simulink model "rtwdemo_dow"  (Simulink 7.6)
settings: Solver=FixedStepDiscrete  StartTime=0.0  StopTime=.001  FixedStep=0.001  RelTol=1e-3
PreLoadFcn:
  | rtwdemo_dow_data
values from neighbouring files (symbols this model uses):
  F1 = 2    [rtwdemo_dow_data.m]
  G1 = 4    [rtwdemo_dow_data.m]
  G2 = 5    [rtwdemo_dow_data.m]
  G3 = 6    [rtwdemo_dow_data.m]
  K1 = 3    [rtwdemo_cgv_init.m]    (also in rtwdemo_dow_data.m)
libraries: rtwdemowidgets x2
Description:
  | Creating a Data Dictionary with the Data Object Wizard
settings Model: Creator=The MathWorks Inc.  ExtModeAutoUpdateStatusClock=off
settings MATStruct: SampleTime=0.001  Offset=0  Priority=[20.0]
settings DataIOCC: SaveOutput=off  SaveTime=off
settings OptimizationCC: InlineParams=on  InlineInvariantSignals=on  StateBitsets=on  DataBitsets=on  UseTempVars=on  EfficientFloat2IntCast=on  EfficientMapNaN2IntZero=off  BufferReusableBoundary=off
settings DebuggingCC: CheckExecutionContextPreStartOutputMsg=on  CheckExecutionContextRuntimeOutputMsg=on  SigSpecEnsureSampleTimeMsg=none  StrictBusMsg=ErrorOnBusTreatedAsVector
settings HardwareCC: ProdIntDivRoundTo=Zero  ProdEndianess=LittleEndian  ProdHWDeviceType=Generic->32-bit Embedded Processor  TargetHWDeviceType=Generic->32-bit Embedded Processor
settings SFSimCC: SimParseCustomCode=off
settings RTWCC: GenerateReport=on  RTWVerbose=off  ProcessScript=grt_make_rtw_hook  LaunchReport=on
settings CodeAppCC: ForceParamTrailComments=on
settings GRTTargetCC: TargetFcnLib=ansi_tfl_tmw.mat

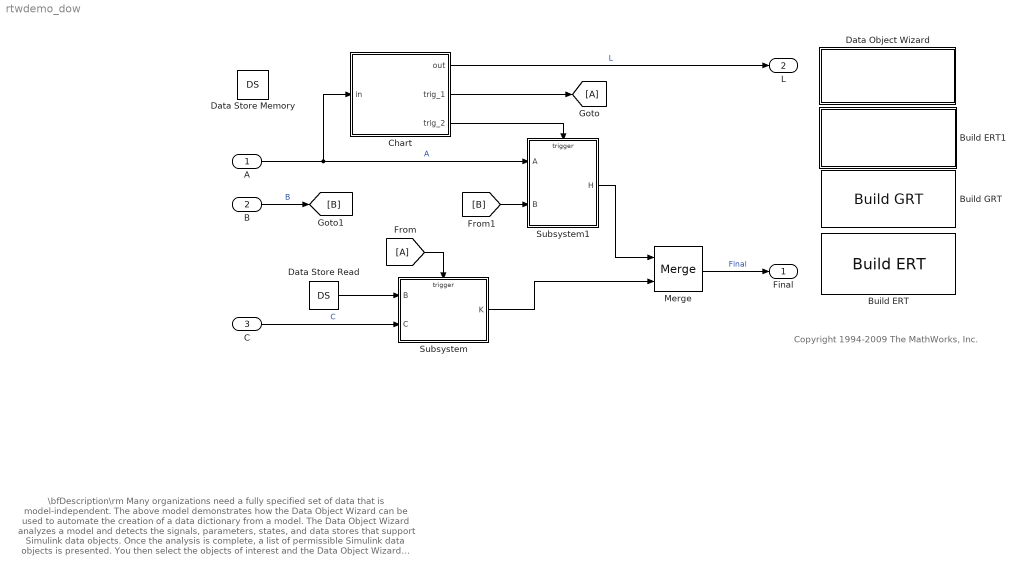
== system rtwdemo_dow ==
  note: \bfDescription\rm
      | Many organizations need a fully specified set of data that is model-independent.  The above model demonstrates how the Data Object Wizard
      | can be used to automate the creation of a data dictionary from a model.  The Data Object Wizard analyzes a model and detects the signals,
      | parameters, states, and data stores that support Simulink data objects.  Once the analysis is complete, a list of permissible Simulink data
      | objects is presented.  You then select the objects of interest and the Data Object Wizard creates the corresponding Simulink data objects.
      |
      | \bfInstructions\rm
      | 1. Double-click the yellow Data Object Wizard button in the upper right of the diagram.
      | 2. Click the Find button to get a list of all signals and parameters that support Simulink Data Objects.
      | 3. Click the Check All button to select all objects.
      | 4. Click the Create button to create the corresponding Simulink data objects.
      | 5. Double-click the yellow Inspect Base Workspace button in the upper right to inspect the data objects.
      | 6. Change the StorageClass of the data objects to ExportedGlobal (batch edit from the spreadsheet view).
      | 7. Generate and inspect the code using the blue buttons in the upper right of the diagram.
      |
      | \bfNotes\rm
      | o  Signals H and K are not presented in the Data Object Wizard because the inputs to the Merge block do not support Simulink data objects.
      |      Only the output of a Merge block  supports data objects.
      | o  Goto and From blocks are supported, as demonstrated by signal B.
      | o  If a MATLAB variable already exists in the base workspace, the Data Object Wizard transfers its value to the Value field of the corresponding
      |     Simulink parameter object.
  note: Copyright 1994-2009 The MathWorks, Inc.
  A : Inport  OutDataTypeStr=double  PortDimensions=1  SampleTime=0.001
  B : Inport  Port=2  OutDataTypeStr=double  PortDimensions=1  SampleTime=0.001
  C : Inport  Port=3  OutDataTypeStr=double  PortDimensions=1  SampleTime=0.001
  Build ERT : rtwdemowidgets/Build ERT  SystemSampleTime=-1  attrib_overrides={}
  Build ERT1 : Subsystem  mask{attrib_overrides={}}
      mask prompts: attrib_overrides "List of attributes to preserve (cell of strings):"
      mask help: Invoke Model Explorer
      settings: OpenFcn=rtwprivate daexplrwsview;
      mask Display:
      | disp(['Inspect Base\nWorkspace\n',...
      | 	  '(double-click)'])
  Build GRT : rtwdemowidgets/Build GRT  SystemSampleTime=-1  attrib_overrides={}
  Chart : Stateflow chart  TreatAsAtomicUnit=on  RTWFcnName=entry_point  RTWFileName=sfcc
      settings: RTWFcnNameOpts=User specified
  Data Object Wizard : Subsystem  Description=DOW
      settings: OpenFcn=dataobjectwizard(bdroot);
      mask Type: Data Object Wizard
      mask Description: Simulink data object wizard for creating potential Simulink data objects.
      mask Help: helpview([docroot,'/toolbox/ecoder/helptargets.map'],'data_obj_wiz');
      mask Display: disp('Data Object\nWizard\n(double-click)')
  Data Store Memory : DataStoreMemory  DataStoreName=DS
  Data Store Read : DataStoreRead  DataStoreName=DS  SampleTime=.001
  Merge : Merge
  Subsystem : Subsystem  TreatAsAtomicUnit=on
  Subsystem1 : Subsystem  TreatAsAtomicUnit=on
  Final : Outport
  L : Outport  Port=2
  wires:
  C/1 -> Subsystem/2(C)  "C"
  A/1 -> Subsystem1/1(A), Chart/1(in)  "A"
  Subsystem1/1(H) -> Merge/1
  Subsystem/1(K) -> Merge/2
  Merge/1 -> Final/1  "Final"
  Chart/3(trig_2) -> Subsystem1/Trigger
  Chart/2(trig_1) -> [A]
  [A] -> Subsystem/Trigger
  Chart/1(out) -> L/1  "L"
  B/1 -> [B]  "B"
  [B] -> Subsystem1/2(B)
  Data Store Read/1 -> Subsystem/1(B)

== system rtwdemo_dow/Build ERT1 ==

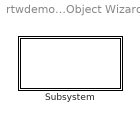
== system rtwdemo_dow/Data Object Wizard ==
  Subsystem : Subsystem

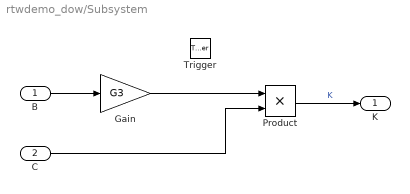
== system rtwdemo_dow/Subsystem ==
  B : Inport
  C : Inport  Port=2
  Trigger : TriggerPort  TriggerType=function-call
  Gain : Gain  Gain=G3
  Product : Product  RndMeth=Zero
  K : Outport
  wires:
  B/1 -> Gain/1
  Gain/1 -> Product/1
  C/1 -> Product/2
  Product/1 -> K/1  "K"

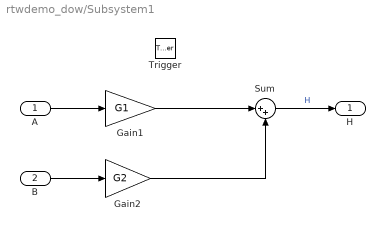
== system rtwdemo_dow/Subsystem1 ==
  A : Inport
  B : Inport  Port=2
  Trigger : TriggerPort  TriggerType=function-call
  Gain1 : Gain  Gain=G1
  Gain2 : Gain  Gain=G2
  Sum : Sum  Inputs=|++
  H : Outport
  wires:
  A/1 -> Gain1/1
  Gain1/1 -> Sum/1
  B/1 -> Gain2/1
  Gain2/1 -> Sum/2
  Sum/1 -> H/1  "H"

== system rtwdemo_dow/Data Object Wizard/Subsystem ==

== stateflow chart Chart ==
  (default) -> (junction 3)
  (junction 3) -> (junction 4) [order 2] : {
      |   out = in;
      |   trig_2;
      | }
  (junction 3) -> (junction 4) [order 1] : [F1 > 10]
      | {
      |   out = in * K1 * G1;
      |   trig_1;
      | }
  data: K1 parameter double; G1 parameter double; in input double; out output double; F1 parameter double
  events: trig_1 output FUNCTION_CALL_EVENT; trig_2 output FUNCTION_CALL_EVENT
